simulink model "power_transient"  (Simulink 6.0)
settings: Solver=ode23tb  SolverMode=SingleTasking  StartTime=0.0  StopTime=0.2  RelTol=1e-3
libraries: powerlib x15
settings Model: Creator=patrice  LastModifiedBy=batserve  ExtModeTrigMode=oneshot  ExtModeArmWhenConnect=off  ExtModeAutoUpdateStatusClock=off
settings DataIOCC: LimitDataPoints=off  SignalLoggingName=sigsOut
settings OptimizationCC: BlockReduction=off  BooleanDataType=off
settings DebuggingCC: CheckExecutionContextPreStartOutputMsg=on  CheckExecutionContextRuntimeOutputMsg=on  SolverPrmCheckMsg=none
settings HardwareCC: TargetUnknown=on
settings RTWCC: TemplateMakefile=grt_unix.tmf

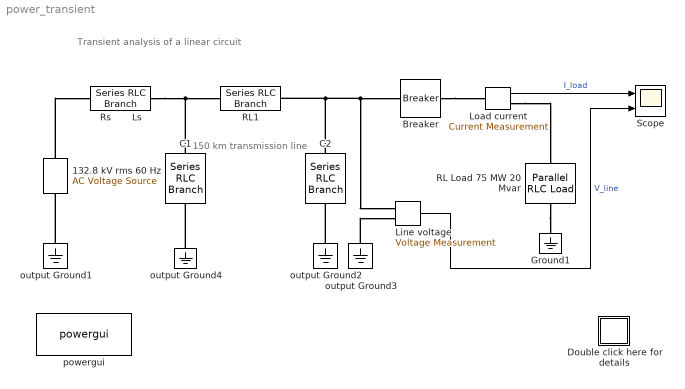
== system power_transient ==
  note: Transient analysis of a linear circuit
  note: 150 km
      | transmission line
  132.8 kV rms 60 Hz : powerlib/Electrical Sources/AC Voltage Source  Description=source block  Orientation=up  Amplitude=230e3/sqrt(3)*sqrt(2)  Phase=90  Frequency=60  SampleTime=0  Measurements=None
      settings: AttributesFormatString=\n
  Breaker : powerlib/Elements/Breaker  BreakerResistance=0.01  InitialState=1  SnubberResistance=inf  SnubberCapacitance=0  SwitchingTimes="[ 2/60  7/60 ]"  External=off  Measurements=None
      settings: AttributesFormatString=\n
  C1 : powerlib/Elements/Series RLC Branch  Orientation=up  PhysicalDomain=powersysdomain  SubClassName=unknown  LeftPortType=p1  RightPortType=p1  LConnTagsString=__new0  RConnTagsString=__new0  Resistance=0  Inductance=0  Capacitance=0.967e-06  Measurements=None
  C2 : powerlib/Elements/Series RLC Branch  Orientation=up  PhysicalDomain=powersysdomain  SubClassName=unknown  LeftPortType=p1  RightPortType=p1  LConnTagsString=__new0  RConnTagsString=__new0  Resistance=0  Inductance=0  Capacitance=0.967e-06  Measurements=None
  Double click here for details : Subsystem
      mask Display: disp('?')
  Ground1 : powerlib/Elements/Ground  Orientation=down  PhysicalDomain=powersysdomain  SubClassName=unknown  LeftPortType=p1  RightPortType=p1  LConnTagsString=a
  Line voltage : powerlib/Measurements/Voltage Measurement  Tag=PoWeRsYsTeMmEaSuReMeNt  PhasorSimulation=off  OutputType=Magnitude  PSBequivalent=0
  Load current : powerlib/Measurements/Current Measurement  Tag=PoWeRsYsTeMmEaSuReMeNt  PhasorSimulation=off  OutputType=Magnitude  PSBequivalent=0
  RL Load 75 MW 20 Mvar : powerlib/Elements/Parallel RLC Load  Orientation=down  PhysicalDomain=powersysdomain  SubClassName=unknown  LeftPortType=p1  RightPortType=p1  LConnTagsString=a  RConnTagsString=__new0  NominalVoltage=132.8e3  NominalFrequency=60  ActivePower=75e6  InductivePower=20e6  CapacitivePower=0  Measurements=None
      settings: AttributesFormatString=\n
  RL1 : powerlib/Elements/Series RLC Branch  PhysicalDomain=powersysdomain  SubClassName=unknown  LeftPortType=p1  RightPortType=p1  LConnTagsString=__new0  RConnTagsString=__new0  Resistance=5.2  Inductance=138e-3  Capacitance=inf  Measurements=None
  Rs       Ls : powerlib/Elements/Series RLC Branch  PhysicalDomain=powersysdomain  SubClassName=unknown  LeftPortType=p1  RightPortType=p1  LConnTagsString=__new0  RConnTagsString=__new0  Resistance=2.645  Inductance=70.2e-03  Capacitance=inf  Measurements=None
  Scope : Scope  NumInputPorts=2
      settings: TimeRange=0.2  YMin=-1000~-400000  YMax=1000~400000  DataFormat=Array
  output Ground{1..4} (4 alike) : powerlib/Elements/Ground  Orientation=down  PhysicalDomain=powersysdomain  SubClassName=unknown  LeftPortType=p1  RightPortType=p1  LConnTagsString=a
  powergui : powerlib/powergui  Priority=2  Frange=logspace(0,3,50)  Ylog=off  Xlog=off  save=off  variable=ZData  ZoomFFT=on  StartTime=0.0  cycles=1  DisplayStyle=off  fundamental=60  FreqAxis=off  MaxFrequency=1000  frequencyindice=1  frequencyindicesteady=1  RmsSteady=1  display=off  Ts=0  methode=off  frequency=60  echomessages=on
  wires:
  Line voltage/1 -> Scope/2  "V_line"
  Load current/1 -> Scope/1  "I_load"
  connections:
  RL Load 75 MW 20 Mvar/RConn1 -- Ground1/LConn1
  output Ground3/LConn1 -- Line voltage/LConn2
  output Ground2/LConn1 -- C2/LConn1
  Line voltage/LConn1 -- Breaker/LConn1 -- RL1/RConn1 -- C2/RConn1
  132.8 kV rms 60 Hz/RConn1 -- Rs       Ls/LConn1
  output Ground1/LConn1 -- 132.8 kV rms 60 Hz/LConn1
  Breaker/RConn1 -- Load current/LConn1
  Load current/RConn1 -- RL Load 75 MW 20 Mvar/LConn1
  Rs       Ls/RConn1 -- RL1/LConn1 -- C1/RConn1
  output Ground4/LConn1 -- C1/LConn1

== system power_transient/Double click here for details ==
  note: This demonstration illustrates steady-state and transient simulation of a linear circuit and use of the Powergui block
  note: Circuit Description
  note: This circuit is a simplified model of a 230 kV three-phase power system. Only one phase of the transmission system is represented.
      | The equivalent source is modeled by a voltage source (230 kV rms/sqrt(3) or 187.8 kV peak, 60 Hz) in series with its  internal impedance (Rs Ls)
      | corresponding to  a 3-phase 2000 MVA short circuit level and X/R = 10. (X = 230e3^2/2000e6 = 26.45 ohms or L = 0.0702 H, R = X/10 = 2.645 ohms).
      | The source feeds a RL load through a 150 km transmission line. The line distributed parameters  (R = 0.035ohm/km, L = 0.92 mH/km, C = 12.9 nF/km)
      |  are modeled by a single pi section (RL1 branch 5.2 ohm; 138 mH  and  two shunt capacitances  C1 and C2 of  0.967 uF).
      | The load (75 MW - 20 Mvar per phase) is modeled by a parallel RLC load block.
      |
      | A circuit breaker is used to switch the load at  the receiving end of the transmission line. The breaker which is initially  closed is opened at t = 2 cycles,
      | then it is reclosed at t = 7 cycles. Current and Voltage Measurement blocks provide signals for visualization purpose.
  note: H. Le-Huy (Universite Laval, Quebec) and G. Sybille (Hydro-Quebec)
  note: Start the simulation and observe  line voltage and  load current  transients during  load switching and note that the simulation starts in steady-state.
      | Use the zoom buttons of the oscilloscope to observe the transient voltage at breaker reclosing.
  note: 1. Simulation using a continuous solver (ode23tb)
  note: Open the Powergui block and select "Steady State Voltage and Currents" to measure the steady-state  voltage and current  phasors.
      |
      | Using the Powergui select now  "Initial  States Setting"  to obtain the initial state values (voltage across capacitors and current in inductances).
      | Now, reset all the initial states to zero by clicking the  "to zero" button and then "Apply" to confirm changes. Restart the simulation and observe transients
      | at simulation starting. Using the same Powergui window, you can also set selected states to specific values.
  note: 2. Using the Powergui to obtain steady-state phasors and set initial states
  note: 3. Discretizing your circuit and simulating at fixed steps
  note: The Powergui block can also be used to  discretize your circuit and simulate it at fixed steps.
      |
      | Open the Powergui. Select  "Discretize electrical model" and specify a sample time of 50e-6 s. The state-space model will now be discretized
      | using trapezoidal fixed step integration. The precision of results is now imposed by the sample time. Restart the simulation and compare simultion results
      | with the continuous integration method.  Vary the sample time of the discrete system and note the impact on precision of fast transients.
  note: 4. Using the phasor simulation method
  note: You will now use a third simulation technique.  The "phasor simulation" method consists to replace the circuit state-space model by a set of algebraic
      | equations evaluated at a fixed frequency and to replace sinusoidal voltage and current sources by phasors (complex numbers). This method allows a fast
      | computation of voltage and current phasors at a selected frequency, disregarding fast transients. It is particularly efficient to study electromechanical
      | transients of generators and motors involving low frequency oscillation modes.
      |
      | Open  the Powergui  block and select "Phasor simulation". Restart the simulation. Observe that the magnitude of 60 Hz  voltage and current is now displayed
      | on the scope. If you double click on the  voltage or current measurement block you can choose to output phasor signals in four different formats:
      | Complex, Real/Imag, Magnitude/Angle (in degres),  or just Magnitude (default value). Notice that you cannot send a complex signal to an oscilloscope.
  note: Demonstration
